simulink model "env_extQ16"  (R2022b)
settings: Solver=VariableStepAuto  StartTime=0.0  StopTime=30  RelTol=1e-3
values from neighbouring files (symbols this model uses):
  B = 8    [variables.m]    (also in variables16.m)
  cordic_delay = 20    [variables.m]    (also in variables16.m)
  e_val = 1/l2    [variables.m]    (also in variables16.m)
  exp_fract_len_homo = 26    [variables.m]    (also in variables16.m = 10)
  exp_word_len_homo = 32    [variables.m]    (also in variables16.m = 16)
  explarge_delay = 3    [variables.m]    (also in variables16.m)
  fft_len_hilb = 2048    [variables.m]    (also in variables16.m)
  fft_length = 4096    [variables.m]    (also in variables16.m)
  frac_bit_l2 = 30    [variables.m]    (also in variables16.m = 14)
  frac_bit_l3 = 29    [variables.m]    (also in variables16.m = 13)
  frac_bit_l4 = 28    [variables.m]    (also in variables16.m = 12)
  grp_delay_hilb = 11    [variables.m]    (also in variables16.m)
  grp_delay_homo = 13    [variables.m]    (also in variables16.m)
  grp_delay_psd = 19    [variables.m]    (also in variables16.m)
  grp_delay_swt = 12    [variables.m]    (also in variables16.m)
  l2 = log(2)    [variables.m]    (also in variables16.m)
  l2e = 1/log2(exp(1))    [variables.m]    (also in variables16.m)
  log2_table = log2((2^(B-1) : 2^(B)) / 2^(B - 1))    [variables.m]    (also in variables16.m)
  log_fract_len_homo = 31    [variables.m]    (also in variables16.m = 15)
  log_latency = 21    [variables.m]    (also in variables16.m)
  log_word_len = 48    [variables.m]    (also in variables16.m = 24)
  log_word_len_homo = 32    [variables.m]    (also in variables16.m = 16)
  NLZLUT = B-ceil(log2((1:2^B)))    [variables.m]    (also in variables16.m)
  scale = 1.0 / (fs * sum(window_val.*window_val))    [variables.m]    (also in variables16.m)
  win_dim = 64    [variables.m]    (also in variables16.m)
  window_dim = 100    [variables.m]    (also in variables16.m)
undefined symbols (not defined in the file or in its folder): C, c, fl_high_index, fl_low_index, HiD, hilbert_fifo_full, LoD, psd_fifo_full, SFVC784, swt_fifo_full, XCK26, xlfda_numerator
libraries: hdlBasic x626, hdlDSPIP x12, hdlUtilities x2, dspsnks4 x1, dspvision x1, vmcUtilities x1
(part 3 of 7)

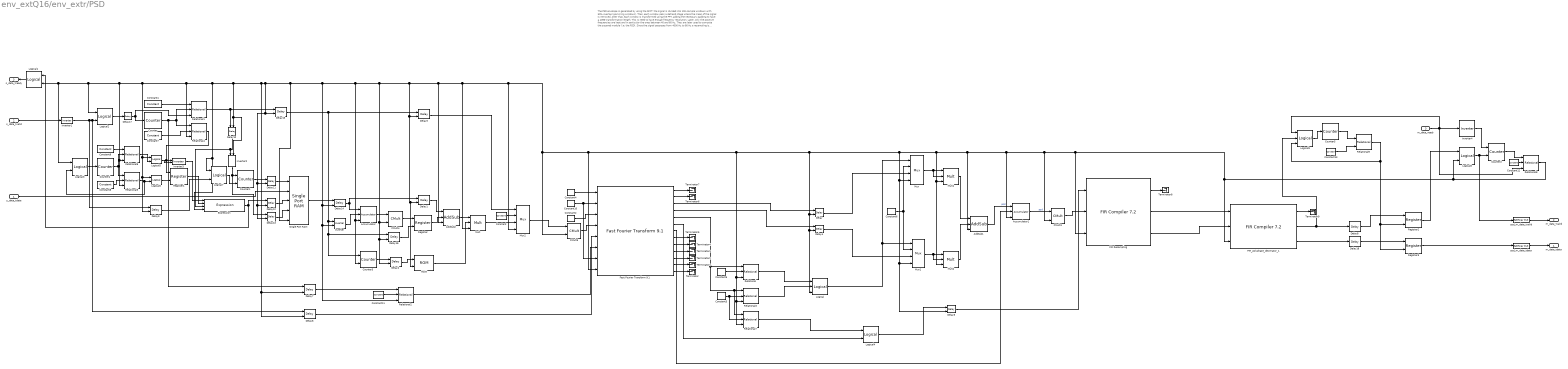
== system env_extQ16/env_extr/PSD ==
  note: The PSD envelope is generated by using the SFFT: the signal is divided into 100-sample windows with 50% overlap (Hamming windows). Then, each window pass a detrend stage where the mean of the signal is removed. After that, each window is transformed using the FFT, adding the necessary padding to have a 4096 transformation length. This is need to have enough frequency resolution.
      | Later, only the positive frequencies are kept and in particular the ones between 40 and 60 Hz. They are later used to compute the squared module (i.e. the PSD).
      | Since the signal passeses from 4000 Hz to 80 Hz a resampling is needed and instead of using a resample method based on FFT, a polyphase interpolator is employed.
      |
      | More at: https://docs.scipy.org/doc/scipy/reference/generated/scipy.signal.spectrogram.html and
      | https://ieeexplore.ieee.org/document/7234876
  s_data_tdata : Inport
  s_data_tvalid : Inport  Port=2
  m_data_ready : Inport  Port=3
  Accumulator : hdlBasic/Accumulator  operation=Add  n_bits=32  overflow=Wrap  scale=1  rst=on  hasbypass=off  en=on  latency=1  msb_inp=100  msb=100  lsb=-100  use_behavioral_HDL=on  implementation=Fabric  XmcBlockStatus=1  maskContainerNames=group3  block_type=accum  block_config=sysgen:Accum_config  block_width=566  block_height=845
  Accumulator1 : hdlBasic/Accumulator  operation=Add  n_bits=64  overflow=Wrap  scale=1  rst=on  hasbypass=off  en=on  latency=1  msb_inp=203  msb=203  lsb=-100  use_behavioral_HDL=on  implementation=Fabric  XmcBlockStatus=1  maskContainerNames=group3  block_type=accum  block_config=sysgen:Accum_config  block_width=566  block_height=845
  AddSub1 : hdlBasic/AddSub  mode=Addition  use_carryin=off  use_carryout=off  en=on  latency=1  precision=User Defined  arith_type="Signed  (2's comp)"  n_bits=32  bin_pt=30  quantization="Round  (unbiased: +/- Inf)"  overflow=Wrap  use_behavioral_HDL=off  hw_selection=Fabric  pipelined=off  XmcBlockStatus=1  maskContainerNames=tabcontainer1  block_type=addsub  block_config=sysgen:Addsub_config
  AddSub2 : hdlBasic/AddSub  mode=Subtraction  use_carryin=off  use_carryout=off  en=on  latency=1  precision=User Defined  arith_type="Signed  (2's comp)"  n_bits=32  bin_pt=31  quantization="Round  (unbiased: +/- Inf)"  overflow=Wrap  use_behavioral_HDL=off  hw_selection=Fabric  pipelined=off  XmcBlockStatus=1  maskContainerNames=tabcontainer1  block_type=addsub  block_config=sysgen:Addsub_config
  CMult3 : hdlBasic/CMult  const=(scale*128*128*2*2)/(fl_high_index-fl_low_index)  gui_display_data_type=Fixed-point  const_n_bits=32  const_bin_pt=31  float_type=Single  exp_bits=8  fraction_bits=24  en=on  latency=1  precision=User Defined  arith_type="Signed  (2's comp)"  n_bits=32  bin_pt=30  quantization="Round  (unbiased: +/- Inf)"  overflow=Wrap  use_behavioral_HDL=off  mem_type=Distributed RAM  pipeline=off  XmcBlockStatus=1  maskContainerNames=tabcontainer1  block_type=cmult  block_config=sysgen:CMult_config
      settings: infoedit=[]
  CMult4 : hdlBasic/CMult  const=1/window_dim  gui_display_data_type=Fixed-point  const_n_bits=32  const_bin_pt=31  float_type=Single  exp_bits=8  fraction_bits=24  en=on  latency=1  precision=User Defined  arith_type="Signed  (2's comp)"  n_bits=32  bin_pt=30  quantization="Round  (unbiased: +/- Inf)"  overflow=Wrap  use_behavioral_HDL=off  mem_type=Distributed RAM  pipeline=off  XmcBlockStatus=1  maskContainerNames=tabcontainer1  block_type=cmult  block_config=sysgen:CMult_config
      settings: infoedit=[]
  CMult5 : hdlBasic/CMult  const=1/128  gui_display_data_type=Fixed-point  const_n_bits=32  const_bin_pt=31  float_type=Single  exp_bits=8  fraction_bits=24  en=on  latency=1  precision=User Defined  arith_type="Signed  (2's comp)"  n_bits=32  bin_pt=31  quantization="Round  (unbiased: +/- Inf)"  overflow=Wrap  use_behavioral_HDL=off  mem_type=Distributed RAM  pipeline=off  XmcBlockStatus=1  maskContainerNames=tabcontainer1  block_type=cmult  block_config=sysgen:CMult_config
      settings: infoedit=[]
  Constant : hdlBasic/Constant  const=0  gui_display_data_type=Fixed-point  arith_type=Signed (2's comp)  n_bits=32  bin_pt=31  preci_type=Single  exp_width=8  frac_width=24  explicit_period=off  period=1  XmcBlockStatus=1  maskContainerNames=tabcontainer1  block_type=constant  block_config=sysgen:Constant_config
  Constant1 : hdlBasic/Constant  const=window_dim  gui_display_data_type=Fixed-point  arith_type=Unsigned  n_bits=ceil(log2(window_dim))  bin_pt=0  preci_type=Single  exp_width=8  frac_width=24  explicit_period=off  period=1  XmcBlockStatus=1  maskContainerNames=tabcontainer1  block_type=constant  block_config=sysgen:Constant_config
  Constant10 : hdlBasic/Constant  const=1.0  gui_display_data_type=Boolean  arith_type=Boolean  n_bits=16  bin_pt=14  preci_type=Single  exp_width=8  frac_width=24  explicit_period=off  period=1  XmcBlockStatus=1  maskContainerNames=tabcontainer1  block_type=constant  block_config=sysgen:Constant_config
  Constant11 : hdlBasic/Constant  const=4094  gui_display_data_type=Fixed-point  arith_type=Unsigned  n_bits=ceil(log2(fft_length))  bin_pt=0  preci_type=Single  exp_width=8  frac_width=24  explicit_period=off  period=1  XmcBlockStatus=1  maskContainerNames=tabcontainer1  block_type=constant  block_config=sysgen:Constant_config
  Constant12 : hdlBasic/Constant  const=win_dim  gui_display_data_type=Fixed-point  arith_type=Unsigned  n_bits=win_bit  bin_pt=0  preci_type=Single  exp_width=8  frac_width=24  explicit_period=off  period=1  XmcBlockStatus=1  maskContainerNames=tabcontainer1  block_type=constant  block_config=sysgen:Constant_config
  Constant13 : hdlBasic/Constant  const=grp_delay_psd  gui_display_data_type=Fixed-point  arith_type=Unsigned  n_bits=ceil(log2(grp_delay_psd))  bin_pt=0  preci_type=Single  exp_width=8  frac_width=24  explicit_period=off  period=1  XmcBlockStatus=1  maskContainerNames=tabcontainer1  block_type=constant  block_config=sysgen:Constant_config
  Constant2 : hdlBasic/Constant  const=0  gui_display_data_type=Fixed-point  arith_type=Signed (2's comp)  n_bits=32  bin_pt=31  preci_type=Single  exp_width=8  frac_width=24  explicit_period=on  period=sample_period_psd  XmcBlockStatus=1  maskContainerNames=tabcontainer1  block_type=constant  block_config=sysgen:Constant_config
  Constant3 : hdlBasic/Constant  const=fl_high_index-1  gui_display_data_type=Fixed-point  arith_type=Unsigned  n_bits=ceil(log2(fl_high_index-1))  bin_pt=0  preci_type=Single  exp_width=8  frac_width=24  explicit_period=off  period=1  XmcBlockStatus=1  maskContainerNames=tabcontainer1  block_type=constant  block_config=sysgen:Constant_config
  Constant4 : hdlBasic/Constant  const=1.0  gui_display_data_type=Fixed-point  arith_type=Unsigned  n_bits=1  bin_pt=0  preci_type=Single  exp_width=8  frac_width=24  explicit_period=off  period=1  XmcBlockStatus=1  maskContainerNames=tabcontainer1  block_type=constant  block_config=sysgen:Constant_config
  Constant5 : hdlBasic/Constant  const=fl_low_index-1  gui_display_data_type=Fixed-point  arith_type=Unsigned  n_bits=ceil(log2(fl_low_index-1))  bin_pt=0  preci_type=Single  exp_width=8  frac_width=24  explicit_period=off  period=1  XmcBlockStatus=1  maskContainerNames=tabcontainer1  block_type=constant  block_config=sysgen:Constant_config
  Constant6 : hdlBasic/Constant  const=0  gui_display_data_type=Fixed-point  arith_type=Signed (2's comp)  n_bits=32  bin_pt=30  preci_type=Single  exp_width=8  frac_width=24  explicit_period=off  period=1  XmcBlockStatus=1  maskContainerNames=tabcontainer1  block_type=constant  block_config=sysgen:Constant_config
  Constant7 : hdlBasic/Constant  const=(window_dim/2)-1  gui_display_data_type=Fixed-point  arith_type=Unsigned  n_bits=ceil(log2((window_dim/2)-1))  bin_pt=0  preci_type=Single  exp_width=8  frac_width=24  explicit_period=off  period=1  XmcBlockStatus=1  maskContainerNames=tabcontainer1  block_type=constant  block_config=sysgen:Constant_config
  Constant8 : hdlBasic/Constant  const=(window_dim/2)  gui_display_data_type=Fixed-point  arith_type=Unsigned  n_bits=ceil(log2((window_dim/2)+2))  bin_pt=0  preci_type=Single  exp_width=8  frac_width=24  explicit_period=off  period=1  XmcBlockStatus=1  maskContainerNames=tabcontainer1  block_type=constant  block_config=sysgen:Constant_config
  Constant9 : hdlBasic/Constant  const=(window_dim/2)-1  gui_display_data_type=Fixed-point  arith_type=Unsigned  n_bits=ceil(log2((window_dim/2)+1))  bin_pt=0  preci_type=Single  exp_width=8  frac_width=24  explicit_period=off  period=1  XmcBlockStatus=1  maskContainerNames=tabcontainer1  block_type=constant  block_config=sysgen:Constant_config
  Counter : hdlBasic/Counter  cnt_type=Free running  cnt_to=4094  operation=Up  start_count=0  cnt_by_val=1  arith_type=Unsigned  n_bits=ceil(log2(fft_length))  bin_pt=0  load_pin=off  rst=off  en=on  explicit_period=Explicit  period=sample_period_psd  use_behavioral_HDL=off  implementation=Fabric  XmcBlockStatus=1  maskContainerNames=group1  block_type=counter  block_config=sysgen:Counter_config  block_width=531  block_height=1023
  Counter1 : hdlBasic/Counter  cnt_type=Count limited  cnt_to=(window_dim/2)-1  operation=Up  start_count=0  cnt_by_val=1  arith_type=Unsigned  n_bits=ceil(log2((window_dim/2)-1))  bin_pt=0  load_pin=off  rst=on  en=on  explicit_period=Explicit  period=sample_period_psd  use_behavioral_HDL=off  implementation=Fabric  XmcBlockStatus=1  maskContainerNames=group1  block_type=counter  block_config=sysgen:Counter_config  block_width=531  block_height=1023
  Counter2 : hdlBasic/Counter  cnt_type=Free running  cnt_to=Inf  operation=Up  start_count=0  cnt_by_val=1  arith_type=Unsigned  n_bits=win_bit  bin_pt=0  load_pin=off  rst=on  en=on  explicit_period=Explicit  period=sample_period_psd  use_behavioral_HDL=off  implementation=Fabric  XmcBlockStatus=1  maskContainerNames=group1  block_type=counter  block_config=sysgen:Counter_config  block_width=531  block_height=1023
  Counter3 : hdlBasic/Counter  cnt_type=Count limited  cnt_to=window_dim-1  operation=Up  start_count=0  cnt_by_val=1  arith_type=Unsigned  n_bits=ceil(log2(window_dim-1))  bin_pt=0  load_pin=off  rst=on  en=on  explicit_period=Explicit  period=sample_period_psd  use_behavioral_HDL=off  implementation=Fabric  XmcBlockStatus=1  maskContainerNames=group1  block_type=counter  block_config=sysgen:Counter_config  block_width=531  block_height=1023
  Counter4 : hdlBasic/Counter  cnt_type=Free running  cnt_to=100  operation=Up  start_count=0  cnt_by_val=1  arith_type=Unsigned  n_bits=7  bin_pt=0  load_pin=off  rst=off  en=on  explicit_period=Explicit  period=sample_period_psd  use_behavioral_HDL=off  implementation=Fabric  XmcBlockStatus=1  maskContainerNames=group1  block_type=counter  block_config=sysgen:Counter_config  block_width=531  block_height=1023
  Counter5 : hdlBasic/Counter  cnt_type=Free running  cnt_to=Inf  operation=Up  start_count=0  cnt_by_val=1  arith_type=Unsigned  n_bits=ceil(log2(grp_delay_psd))  bin_pt=0  load_pin=off  rst=off  en=on  explicit_period=Explicit  period=sample_period_psd  use_behavioral_HDL=off  implementation=Fabric  XmcBlockStatus=1  maskContainerNames=group1  block_type=counter  block_config=sysgen:Counter_config  block_width=531  block_height=1023
  Delay : hdlBasic/Delay  rst=off  en=on  latency=2  reg_retiming=off  XmcBlockStatus=1  maskContainerNames=group1  block_type=delay  block_config=sysgen:Delay_config
  Delay1 : hdlBasic/Delay  rst=off  en=on  latency=window_dim+2  reg_retiming=off  XmcBlockStatus=1  maskContainerNames=group1  block_type=delay  block_config=sysgen:Delay_config
  Delay{10..14} (5 alike) : hdlBasic/Delay  rst=off  en=on  latency=1  reg_retiming=off  XmcBlockStatus=1  maskContainerNames=group1  block_type=delay  block_config=sysgen:Delay_config
  Delay15 : hdlBasic/Delay  rst=off  en=on  latency=4  reg_retiming=off  XmcBlockStatus=1  maskContainerNames=group1  block_type=delay  block_config=sysgen:Delay_config
  Delay16 : hdlBasic/Delay  rst=off  en=on  latency=3  reg_retiming=off  XmcBlockStatus=1  maskContainerNames=group1  block_type=delay  block_config=sysgen:Delay_config
  Delay17 : hdlBasic/Delay  rst=off  en=off  latency=1  reg_retiming=off  XmcBlockStatus=1  maskContainerNames=group1  block_type=delay  block_config=sysgen:Delay_config
  Delay18 : hdlBasic/Delay  rst=off  en=off  latency=1  reg_retiming=off  XmcBlockStatus=1  maskContainerNames=group1  block_type=delay  block_config=sysgen:Delay_config
  Delay2 : hdlBasic/Delay  rst=off  en=on  latency=3  reg_retiming=off  XmcBlockStatus=1  maskContainerNames=group1  block_type=delay  block_config=sysgen:Delay_config
  Delay3 : hdlBasic/Delay  rst=off  en=on  latency=window_dim+7  reg_retiming=off  XmcBlockStatus=1  maskContainerNames=group1  block_type=delay  block_config=sysgen:Delay_config
  Delay4 : hdlBasic/Delay  rst=off  en=on  latency=2  reg_retiming=off  XmcBlockStatus=1  maskContainerNames=group1  block_type=delay  block_config=sysgen:Delay_config
  Delay5 : hdlBasic/Delay  rst=off  en=on  latency=8  reg_retiming=off  XmcBlockStatus=1  maskContainerNames=group1  block_type=delay  block_config=sysgen:Delay_config
  Delay6 : hdlBasic/Delay  rst=off  en=on  latency=114  reg_retiming=off  XmcBlockStatus=1  maskContainerNames=group1  block_type=delay  block_config=sysgen:Delay_config
  Delay7 : hdlBasic/Delay  rst=off  en=on  latency=113  reg_retiming=off  XmcBlockStatus=1  maskContainerNames=group1  block_type=delay  block_config=sysgen:Delay_config
  Delay8 : hdlBasic/Delay  rst=off  en=off  latency=1  reg_retiming=off  XmcBlockStatus=1  maskContainerNames=group1  block_type=delay  block_config=sysgen:Delay_config
  Delay9 : hdlBasic/Delay  rst=off  en=on  latency=3  reg_retiming=off  XmcBlockStatus=1  maskContainerNames=group1  block_type=delay  block_config=sysgen:Delay_config
  Expression : hdlBasic/Expression  expression=~(a ^ b) & c  align_bp=on  en=on  latency=1  precision=Full  arith_type=Unsigned  n_bits=16  bin_pt=0  XmcBlockStatus=1  maskContainerNames=tabcontainer1  block_type=expr  block_config=sysgen:Expr_config
  FIR Resampling : hdlDSPIP/FIR Compiler 7.2   coefficientvector=fir_interpolator.Numerator  coefficient_sets=1  coefficient_reload=off  filter_type=Interpolation  rate_change_type=Integer  interpolation_rate=50  decimation_rate=1  zero_pack_factor=1  channel_sequence=Basic  number_channels=1  pattern_list='P4-0,P4-1,P4-2,P4-3,P4-4'  number_paths=1  ratespecification=Input_Sample_Period  sampleperiod=fft_length  hardwareoversamplingrate=1  coefficient_sign=Signed  quantization=Quantize_Only  coefficient_width=coeff_width  bestprecision=on  coefficient_fractional_bits=30  coefficient_structure=Non_Symmetric  output_rounding_mode=Convergent_Rounding_to_Even  output_width=output_width  filter_architecture=Systolic_Multiply_Accumulate  optimization_goal=Area  optimization_list='None'  data_buffer_type=Automatic  coefficient_buffer_type=Automatic  input_buffer_type=Automatic  output_buffer_type=Automatic  preference_for_other_storage=Automatic  multi_column_support=Automatic  columnconfig='1'  inter_column_pipe_length=4  data_has_tlast=Not_Required  m_data_has_tready=off  s_data_has_fifo=off  s_data_has_tuser=Not_Required  m_data_has_tuser=Not_Required  s_config_sync_mode=On_Vector  s_config_method=Single  num_reload_slots=1  has_aclken=on  has_aresetn=off  reset_data_vector=on  trim_axipin_name=off  simulation_type=hybrid_sim  simulation_model=sysgen:xfirv7_2_cmodel  data_path_portlist={ 's_axis_data_tdata', 'm_axis_data_tdata' }  passband_min=0.0  passband_max=0.5  stopband_min=0.5  stopband_max=1.0  filter_selection=1  gui_behaviour='Sysgen_GUI'  data_sign=Signed  data_width=16  data_fractional_bits=0  data_tuser_width=1  wrapper_available=true  ip_wrap_arbitrary_binary_point=true  ip_name=FIR Compiler  ip_version=7.2  dsptool_ready=true  ipcore_usecache=true  ipcore_useipmodelcache=true  port_translation_map={ 'aclken' => 'en', 'aresetn' => 'rst' }  run_core_at_system_period=true  ipcore_xco_need_fpga_part=true  ipcore_fpga_part=[]  XmcBlockStatus=1  maskContainerNames=tabcontainer1  block_type=fir_compiler_v7_2  block_config=sysgen:rodinimport_config  block_width=820  block_height=600
  FIR_polyphase_decimator_1 : hdlDSPIP/FIR Compiler 7.2   coefficientvector=firdecim.Numerator  coefficient_sets=1  coefficient_reload=off  filter_type=Decimation  rate_change_type=Integer  interpolation_rate=1  decimation_rate=80  zero_pack_factor=1  channel_sequence=Basic  number_channels=1  pattern_list='P4-0,P4-1,P4-2,P4-3,P4-4'  number_paths=1  ratespecification=Input_Sample_Period  sampleperiod=1  hardwareoversamplingrate=1  coefficient_sign=Signed  quantization=Quantize_Only  coefficient_width=coeff_width  bestprecision=on  coefficient_fractional_bits=37  coefficient_structure=Non_Symmetric  output_rounding_mode=Convergent_Rounding_to_Even  output_width=output_width  filter_architecture=Systolic_Multiply_Accumulate  optimization_goal=Area  optimization_list='None'  data_buffer_type=Automatic  coefficient_buffer_type=Automatic  input_buffer_type=Automatic  output_buffer_type=Automatic  preference_for_other_storage=Automatic  multi_column_support=Automatic  columnconfig='24'  inter_column_pipe_length=4  data_has_tlast=Not_Required  m_data_has_tready=off  s_data_has_fifo=off  s_data_has_tuser=Not_Required  m_data_has_tuser=Not_Required  s_config_sync_mode=On_Vector  s_config_method=Single  num_reload_slots=1  has_aclken=on  has_aresetn=off  reset_data_vector=on  trim_axipin_name=off  simulation_type=hybrid_sim  simulation_model=sysgen:xfirv7_2_cmodel  data_path_portlist={ 's_axis_data_tdata', 'm_axis_data_tdata' }  passband_min=0.0  passband_max=0.5  stopband_min=0.5  stopband_max=1.0  filter_selection=1  gui_behaviour='Sysgen_GUI'  data_sign=Signed  data_width=16  data_fractional_bits=0  data_tuser_width=1  wrapper_available=true  ip_wrap_arbitrary_binary_point=true  ip_name=FIR Compiler  ip_version=7.2  dsptool_ready=true  ipcore_usecache=true  ipcore_useipmodelcache=true  port_translation_map={ 'aclken' => 'en', 'aresetn' => 'rst' }  run_core_at_system_period=true  ipcore_xco_need_fpga_part=true  ipcore_fpga_part=[]  XmcBlockStatus=1  maskContainerNames=tabcontainer1  block_type=fir_compiler_v7_2  block_config=sysgen:rodinimport_config  block_width=820  block_height=600
  Fast Fourier Transform 9.1 : hdlDSPIP/Fast Fourier Transform 9.1   transform_length=4096  target_clock_frequency=fft_freq_psd  target_data_throughput=50  implementation_options=pipelined_streaming_io  run_time_configurable_transform_length=off  phase_factor_width=32  scaling_options=unscaled  rounding_modes=convergent_rounding  aclken=on  aresetn=off  output_ordering=natural_order  cyclic_prefix_insertion=off  throttle_scheme=nonrealtime  xk_index=on  ovflo=off  trim_axipin_name=off  memory_options_data=block_ram  memory_options_phase_factors=block_ram  number_of_stages_using_block_ram_for_data_and_phase_factors=6  memory_options_reorder=block_ram  memory_options_hybrid=off  complex_mult_type=use_mults_resources  butterfly_type=use_luts  simulation_type=hybrid_sim  simulation_model=sysgen:xfftv9_cmodel  data_path_portlist={ 's_axis_data_tdata', 'm_axis_data_tdata', 'm_axis_status_tdata', 'event_fft_overflow' }  channels=1  input_ordering=natural_order  input_width=16  ip_name=Fast Fourier Transform  ip_version=9.1  dsptool_ready=true  ipcore_usecache=true  ipcore_useipmodelcache=true  wrapper_available=true  port_translation_map={ 'aclken' => 'en', 'aresetn' => 'rst'}  data_format=fixed_point  XmcBlockStatus=1  maskContainerNames=tabcontainer1  block_type=xfft_v9_1  block_config=sysgen:rodinimport_config
  Inverter : hdlBasic/Inverter  en=on  latency=1  XmcBlockStatus=1  maskContainerNames=group2  block_type=inv  block_config=sysgen:Inverter_config
  Inverter1 : hdlBasic/Inverter  en=off  latency=0  XmcBlockStatus=1  maskContainerNames=group2  block_type=inv  block_config=sysgen:Inverter_config
  Inverter2 : hdlBasic/Inverter  en=on  latency=1  XmcBlockStatus=1  maskContainerNames=group2  block_type=inv  block_config=sysgen:Inverter_config
  Inverter3 : hdlBasic/Inverter  en=on  latency=1  XmcBlockStatus=1  maskContainerNames=group2  block_type=inv  block_config=sysgen:Inverter_config
  Inverter4 : hdlBasic/Inverter  en=off  latency=0  XmcBlockStatus=1  maskContainerNames=group2  block_type=inv  block_config=sysgen:Inverter_config
  Logical : hdlBasic/Logical  logical_function=AND  inputs=2  en=on  latency=1  precision=Full  arith_type=Unsigned  n_bits=16  bin_pt=0  align_bp=on  overflow=[]  quantization=[]  XmcBlockStatus=1  maskContainerNames=tabcontainer1  block_type=logical  block_config=sysgen:Logical_config
  Logical{1..8} (8 alike) : hdlBasic/Logical  logical_function=AND  inputs=2  en=off  latency=0  precision=Full  arith_type=Unsigned  n_bits=16  bin_pt=0  align_bp=on  overflow=[]  quantization=[]  XmcBlockStatus=1  maskContainerNames=tabcontainer1  block_type=logical  block_config=sysgen:Logical_config
  Logical9 : hdlBasic/Logical  logical_function=AND  inputs=3  en=off  latency=0  precision=Full  arith_type=Unsigned  n_bits=16  bin_pt=0  align_bp=on  overflow=[]  quantization=[]  XmcBlockStatus=1  maskContainerNames=tabcontainer1  block_type=logical  block_config=sysgen:Logical_config
  Mult : hdlBasic/Mult  precision=User Defined  arith_type="Signed  (2's comp)"  n_bits=32  bin_pt=31  quantization="Round  (unbiased: +/- Inf)"  overflow=Wrap  en=on  latency=3  use_behavioral_HDL=off  opt=Speed  use_embedded=on  optimum_pipeline=off  pipeline=on  use_rpm=on  placement_style=Triangular  XmcBlockStatus=1  maskContainerNames=group1  block_type=mult  block_config=sysgen:Mult_config  block_width=598  block_height=876
  Mult1 : hdlBasic/Mult  precision=User Defined  arith_type="Signed  (2's comp)"  n_bits=32  bin_pt=30  quantization="Round  (unbiased: +/- Inf)"  overflow=Wrap  en=on  latency=3  use_behavioral_HDL=off  opt=Speed  use_embedded=on  optimum_pipeline=off  pipeline=on  use_rpm=on  placement_style=Triangular  XmcBlockStatus=1  maskContainerNames=group1  block_type=mult  block_config=sysgen:Mult_config  block_width=598  block_height=876
  Mult2 : hdlBasic/Mult  precision=User Defined  arith_type="Signed  (2's comp)"  n_bits=32  bin_pt=30  quantization="Round  (unbiased: +/- Inf)"  overflow=Wrap  en=on  latency=3  use_behavioral_HDL=off  opt=Speed  use_embedded=on  optimum_pipeline=off  pipeline=on  use_rpm=on  placement_style=Triangular  XmcBlockStatus=1  maskContainerNames=group1  block_type=mult  block_config=sysgen:Mult_config  block_width=598  block_height=876
  Mux : hdlBasic/Mux  inputs=2  en=on  latency=1  precision=Full  arith_type=Unsigned  n_bits=16  bin_pt=14  quantization=Truncate  overflow=Wrap  XmcBlockStatus=1  maskContainerNames=tabcontainer1  block_type=mux  block_config=sysgen:Mux_config
  Mux1 : hdlBasic/Mux  inputs=2  en=on  latency=1  precision=Full  arith_type=Unsigned  n_bits=16  bin_pt=14  quantization=Truncate  overflow=Wrap  XmcBlockStatus=1  maskContainerNames=tabcontainer1  block_type=mux  block_config=sysgen:Mux_config
  Mux2 : hdlBasic/Mux  inputs=2  en=on  latency=1  precision=Full  arith_type="Signed  (2's comp)"  n_bits=32  bin_pt=28  quantization="Round  (unbiased: +/- Inf)"  overflow=Wrap  XmcBlockStatus=1  maskContainerNames=tabcontainer1  block_type=mux  block_config=sysgen:Mux_config
  ROM : hdlBasic/ROM  depth=window_dim  initVector=window_val  distributed_mem=Block RAM  rst=off  init_reg=0  en=on  latency=1  gui_display_data_type=Fixed-point  arith_type="Signed  (2's comp)"  n_bits=32  bin_pt=31  preci_type=Single  exp_width=8  frac_width=24  optimize=Area  use_rpm=on  simulation_type=fast_sim  XmcBlockStatus=1  maskContainerNames=tabcontainer1  block_type=sprom  block_config=sysgen:SPROM_config
  Register : hdlBasic/Register  init=0  rst=off  en=on  XmcBlockStatus=1  maskContainerNames=tabcontainer1  block_type=register  block_config=sysgen:Register_config
  Register1 : hdlBasic/Register  init=0  rst=off  en=on  XmcBlockStatus=1  maskContainerNames=tabcontainer1  block_type=register  block_config=sysgen:Register_config
  Register2 : hdlBasic/Register  init=0  rst=on  en=off  XmcBlockStatus=1  maskContainerNames=tabcontainer1  block_type=register  block_config=sysgen:Register_config
  Register3 : hdlBasic/Register  init=0  rst=on  en=off  XmcBlockStatus=1  maskContainerNames=tabcontainer1  block_type=register  block_config=sysgen:Register_config
  Relational : hdlBasic/Relational  mode=a>=b  op_type=Bool  en=on  latency=1  XmcBlockStatus=1  maskContainerNames=tabcontainer1  block_type=relational  block_config=sysgen:Relational_config
  Relational1 : hdlBasic/Relational  mode=a>b  op_type=Bool  en=on  latency=1  XmcBlockStatus=1  maskContainerNames=tabcontainer1  block_type=relational  block_config=sysgen:Relational_config
  Relational2 : hdlBasic/Relational  mode=a=b  op_type=Bool  en=on  latency=1  XmcBlockStatus=1  maskContainerNames=tabcontainer1  block_type=relational  block_config=sysgen:Relational_config
  Relational3 : hdlBasic/Relational  mode=a<=b  op_type=Bool  en=on  latency=1  XmcBlockStatus=1  maskContainerNames=tabcontainer1  block_type=relational  block_config=sysgen:Relational_config
  Relational4 : hdlBasic/Relational  mode=a>b  op_type=Bool  en=on  latency=1  XmcBlockStatus=1  maskContainerNames=tabcontainer1  block_type=relational  block_config=sysgen:Relational_config
  Relational5 : hdlBasic/Relational  mode=a<b  op_type=Bool  en=on  latency=1  XmcBlockStatus=1  maskContainerNames=tabcontainer1  block_type=relational  block_config=sysgen:Relational_config
  Relational6 : hdlBasic/Relational  mode=a<b  op_type=Bool  en=on  latency=1  XmcBlockStatus=1  maskContainerNames=tabcontainer1  block_type=relational  block_config=sysgen:Relational_config
  Relational7 : hdlBasic/Relational  mode=a=b  op_type=Bool  en=on  latency=1  XmcBlockStatus=1  maskContainerNames=tabcontainer1  block_type=relational  block_config=sysgen:Relational_config
  Relational8 : hdlBasic/Relational  mode=a<b  op_type=Bool  en=on  latency=1  XmcBlockStatus=1  maskContainerNames=tabcontainer1  block_type=relational  block_config=sysgen:Relational_config
  Relational9 : hdlBasic/Relational  mode=a<b  op_type=Bool  en=off  latency=0  XmcBlockStatus=1  maskContainerNames=tabcontainer1  block_type=relational  block_config=sysgen:Relational_config
  Single Port RAM : hdlBasic/Single Port RAM  depth=window_dim/2  initVector=zeros(1,window_dim/2)  distributed_mem=Block RAM  write_mode=Read After Write  rst=on  init_reg=0  en=on  optimize_latency=off  latency=1  optimize=Area  dbl_ovrd=off  simulation_type=fast_sim  XmcBlockStatus=1  maskContainerNames=tabcontainer1  block_type=spram  block_config=sysgen:SPRAM_config
  Terminator{,1..9} (10 alike) : Terminator
  psd_m_data_tdata : hdlBasic/Gateway Out  inherit_from_input=off  hdl_port=on  rows=1  columns=1  UseAsDAC=off  DACChannel='1'  interface=None  automatic_assignment=on  address_offset=hex2dec('00')  intf_name=''  intf_description=''  timing_constraint=None  locs_specified=off  LOCs={}  io_standard={}  XmcBlockStatus=1  maskContainerNames=group4  block_type=gatewayout  block_config=sysgen:gateway_out_config  block_width_w=590  block_height_w=620  block_width=620  block_height=750
  psd_m_data_tvalid : hdlBasic/Gateway Out  inherit_from_input=off  hdl_port=on  rows=1  columns=1  UseAsDAC=off  DACChannel='1'  interface=None  automatic_assignment=on  address_offset=hex2dec('00')  intf_name=''  intf_description=''  timing_constraint=None  locs_specified=off  LOCs={}  io_standard={}  XmcBlockStatus=1  maskContainerNames=group4  block_type=gatewayout  block_config=sysgen:gateway_out_config  block_width_w=590  block_height_w=620  block_width=620  block_height=750
  m_data_tdata : Outport
  m_data_tvalid : Outport  Port=2
  s_data_tready : Outport  Port=3
  wires:
  Constant1/1 -> Relational1/1
  Mult/1 -> Mux2/3
  Constant8/1 -> Relational5/2
  Counter4/1 -> Relational6/2, Relational5/1
  Counter1/1 -> Delay11/1
  Accumulator1/1 -> CMult3/1  "psd"
  Delay2/1 -> ROM/1
  Relational/1 -> Logical/1
  Delay13/1 -> Single Port RAM/4
  Accumulator/1 -> CMult4/1
  Delay16/1 -> Register/2
  Delay10/1 -> Expression/3, Inverter2/1
  Counter3/1 -> Delay2/1
  Delay14/1 -> Delay1/1, Accumulator/1
  Single Port RAM/1 -> Delay14/1
  Relational1/1 -> Delay15/1, Delay10/1
  Inverter3/1 -> Expression/1
  Constant/1 -> Mux2/2
  Delay3/1 -> Mux2/1
  Delay15/1 -> Delay3/1, Counter3/1, Delay16/1, Inverter/1
  Constant6/1 -> Mux1/2, Mux/2
  CMult4/1 -> Register/1
  Mux2/1 -> CMult5/1
  Inverter/1 -> Accumulator/2
  Constant9/1 -> Relational6/1
  Delay11/1 -> Single Port RAM/1
  Register1/1 -> Expression/2
  Constant7/1 -> Relational4/2
  Inverter2/1 -> Delay13/1, Counter1/1
  Relational4/1 -> Register1/1, Inverter3/1
  Expression/1 -> Delay12/1, Logical1/1
  AddSub2/1 -> Mult/1
  s_data_tdata/1 -> Single Port RAM/2
  Constant3/1 -> Relational7/2, Relational3/2
  s_data_tvalid/1 -> Inverter1/1
  Constant5/1 -> Relational/2
  Delay/1 -> Mux/3
  Mult1/1 -> AddSub1/1
  ROM/1 -> Mult/2
  Inverter1/1 -> Delay9/1, Delay6/1, Logical2/2
  Relational5/1 -> Logical6/2, Logical3/2
  Logical/1 -> Mux/1, Mux1/1
  Mult2/1 -> AddSub1/2
  Delay5/1 -> FIR Resampling/1
  Fast Fourier Transform 9.1/5 -> Relational/1, Relational7/1, Relational3/1
  Mux/1 -> Mult1/2, Mult1/1
  Delay4/1 -> Mux1/3
  Counter/1 -> Delay7/1, Relational4/1, Relational1/2
  Register/1 -> AddSub2/2
  AddSub1/1 -> Accumulator1/1  "psd"
  Delay1/1 -> AddSub2/1
  Mux1/1 -> Mult2/2, Mult2/1
  Relational3/1 -> Logical/2
  psd_m_data_tdata/1 -> m_data_tdata/1
  FIR Resampling/3 -> FIR_polyphase_decimator_1/2
  Fast Fourier Transform 9.1/13 -> Terminator/1
  Fast Fourier Transform 9.1/12 -> Terminator1/1
  Fast Fourier Transform 9.1/11 -> Terminator2/1
  Fast Fourier Transform 9.1/10 -> Terminator3/1
  Fast Fourier Transform 9.1/9 -> Terminator4/1
  Fast Fourier Transform 9.1/8 -> Terminator5/1
  Fast Fourier Transform 9.1/1 -> Terminator7/1
  Constant4/1 -> Fast Fourier Transform 9.1/1
  Constant10/1 -> Fast Fourier Transform 9.1/7, Fast Fourier Transform 9.1/2
  Constant2/1 -> Fast Fourier Transform 9.1/3
  Fast Fourier Transform 9.1/7 -> Accumulator1/2
  Fast Fourier Transform 9.1/3 -> Delay/1
  Fast Fourier Transform 9.1/4 -> Delay4/1
  CMult5/1 -> Fast Fourier Transform 9.1/4
  Logical1/1 -> s_data_tready/1
  Fast Fourier Transform 9.1/2 -> Terminator6/1
  Logical2/1 -> Delay17/1
  Logical3/1 -> Counter4/1
  Relational2/1 -> Fast Fourier Transform 9.1/6
  Constant11/1 -> Relational2/2
  Delay6/1 -> Fast Fourier Transform 9.1/5
  Delay7/1 -> Relational2/1
  Fast Fourier Transform 9.1/6 -> Logical4/2
  Logical4/1 -> Delay5/1
  Relational7/1 -> Logical4/1
  CMult3/1 -> FIR Resampling/2
  FIR Resampling/2 -> FIR_polyphase_decimator_1/1
  m_data_ready/1 -> Logical9/1, Relational8/3, Inverter4/1
  Delay9/1 -> Logical7/2
  Logical7/1 -> Counter1/2
  FIR Resampling/1 -> Terminator8/1
  FIR_polyphase_decimator_1/1 -> Terminator9/1
  Logical5/1 -> Inverter3/2
  Relational6/1 -> Logical5/2
  Logical6/1 -> Register1/2
  Delay17/1 -> Relational1/3, Counter/1
  Counter2/1 -> Relational8/1
  Constant12/1 -> Relational8/2
  Inverter4/1 -> Counter2/1
  Logical8/1 -> psd_m_data_tvalid/1, Counter2/2
  psd_m_data_tvalid/1 -> m_data_tvalid/1
  Relational8/1 -> FIR_polyphase_decimator_1/3, FIR Resampling/3, CMult3/2, Accumulator1/3, AddSub1/3, Mult2/3, Mult1/3, Delay5/2, Mux1/4, Mux/4, Logical/3, Delay4/2, Delay/2, Mux2/4, Mult/3, AddSub2/3, ROM/2, Delay1/2, Delay3/2, Delay2/2, Delay16/2, CMult4/2, Counter3/2, Accumulator/3, Relational2/3, Inverter/2, Delay14/2, Single Port RAM/5, Delay13/2, Delay12/2, Delay11/2, Delay15/2, Inverter2/2, Delay10/2, Logical7/1, Expression/4, Relational4/3, Logical5/1, Logical6/1, Delay9/2, Logical2/1, Logical3/1, Logical1/2, Relational5/3, Relational6/3, Delay6/2, Delay7/2, CMult5/2, Fast Fourier Transform 9.1/8, Relational3/3, Relational7/3, Relational/3, Logical8/2
  Delay12/1 -> Single Port RAM/3
  Counter5/1 -> Relational9/1
  Logical9/1 -> Counter5/1
  Relational9/1 -> Logical9/3, Register3/2, Register2/2
  Constant13/1 -> Relational9/2
  FIR_polyphase_decimator_1/3 -> Delay18/1
  FIR_polyphase_decimator_1/2 -> Logical9/2, Delay8/1
  Delay8/1 -> Register2/1
  Delay18/1 -> Register3/1
  Register2/1 -> Logical8/1
  Register3/1 -> psd_m_data_tdata/1

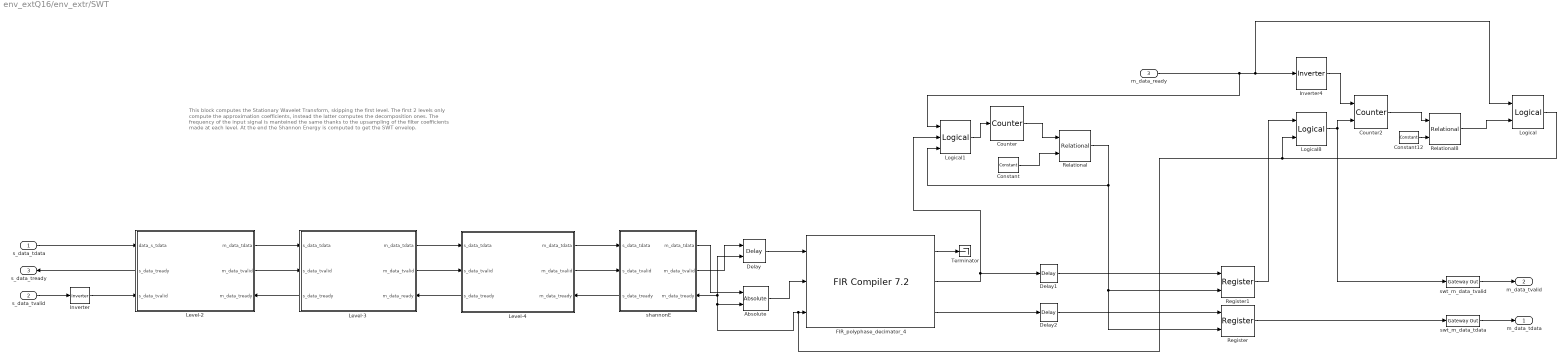
== system env_extQ16/env_extr/SWT ==
  note: This block computes the Stationary Wavelet Transform, skipping the first level. The first 2 levels only compute the approximation coefficients, instead the latter computes the decomposition ones.
      | The frequency of the input signal is manteined the same thanks to the upsampling of the filter coefficients made at each level. At the end the Shannon Energy is computed to get the SWT envelop.
  s_data_tdata : Inport
  s_data_tvalid : Inport  Port=2
  m_data_ready : Inport  Port=3
  Absolute : hdlBasic/Absolute  precision=User Defined  arith_type="Signed  (2's comp)"  n_bits=32  bin_pt=25  quantization="Round  (unbiased: +/- Inf)"  overflow=Saturate  en=on  latency=1  XmcBlockStatus=1  maskContainerNames=tabcontainer1  block_type=abs  block_config=sysgen:Abs_config
  Constant : hdlBasic/Constant  const=grp_delay_swt  gui_display_data_type=Fixed-point  arith_type=Unsigned  n_bits=ceil(log2(grp_delay_swt))  bin_pt=0  preci_type=Single  exp_width=8  frac_width=24  explicit_period=off  period=1  XmcBlockStatus=1  maskContainerNames=tabcontainer1  block_type=constant  block_config=sysgen:Constant_config
  Constant12 : hdlBasic/Constant  const=win_dim  gui_display_data_type=Fixed-point  arith_type=Unsigned  n_bits=win_bit  bin_pt=0  preci_type=Single  exp_width=8  frac_width=24  explicit_period=off  period=1  XmcBlockStatus=1  maskContainerNames=tabcontainer1  block_type=constant  block_config=sysgen:Constant_config
  Counter : hdlBasic/Counter  cnt_type=Free running  cnt_to=Inf  operation=Up  start_count=0  cnt_by_val=1  arith_type=Unsigned  n_bits=ceil(log2(grp_delay_swt))  bin_pt=0  load_pin=off  rst=off  en=on  explicit_period=Explicit  period=sample_period_swt  use_behavioral_HDL=off  implementation=Fabric  XmcBlockStatus=1  maskContainerNames=group1  block_type=counter  block_config=sysgen:Counter_config  block_width=531  block_height=1023
  Counter2 : hdlBasic/Counter  cnt_type=Free running  cnt_to=Inf  operation=Up  start_count=0  cnt_by_val=1  arith_type=Unsigned  n_bits=win_bit  bin_pt=0  load_pin=off  rst=on  en=on  explicit_period=Explicit  period=sample_period_swt  use_behavioral_HDL=off  implementation=Fabric  XmcBlockStatus=1  maskContainerNames=group1  block_type=counter  block_config=sysgen:Counter_config  block_width=531  block_height=1023
  Delay : hdlBasic/Delay  rst=off  en=on  latency=1  reg_retiming=off  XmcBlockStatus=1  maskContainerNames=group1  block_type=delay  block_config=sysgen:Delay_config
  Delay1 : hdlBasic/Delay  rst=off  en=off  latency=1  reg_retiming=off  XmcBlockStatus=1  maskContainerNames=group1  block_type=delay  block_config=sysgen:Delay_config
  Delay2 : hdlBasic/Delay  rst=off  en=off  latency=1  reg_retiming=off  XmcBlockStatus=1  maskContainerNames=group1  block_type=delay  block_config=sysgen:Delay_config
  FIR_polyphase_decimator_4 : hdlDSPIP/FIR Compiler 7.2   coefficientvector=firdecim.Numerator  coefficient_sets=1  coefficient_reload=off  filter_type=Decimation  rate_change_type=Integer  interpolation_rate=1  decimation_rate=80  zero_pack_factor=1  channel_sequence=Basic  number_channels=1  pattern_list='P4-0,P4-1,P4-2,P4-3,P4-4'  number_paths=1  ratespecification=Input_Sample_Period  sampleperiod=1  hardwareoversamplingrate=1  coefficient_sign=Signed  quantization=Quantize_Only  coefficient_width=coeff_width  bestprecision=on  coefficient_fractional_bits=21  coefficient_structure=Non_Symmetric  output_rounding_mode=Convergent_Rounding_to_Even  output_width=output_width  filter_architecture=Systolic_Multiply_Accumulate  optimization_goal=Area  optimization_list='None'  data_buffer_type=Automatic  coefficient_buffer_type=Automatic  input_buffer_type=Automatic  output_buffer_type=Automatic  preference_for_other_storage=Automatic  multi_column_support=Automatic  columnconfig='24'  inter_column_pipe_length=4  data_has_tlast=Not_Required  m_data_has_tready=off  s_data_has_fifo=off  s_data_has_tuser=Not_Required  m_data_has_tuser=Not_Required  s_config_sync_mode=On_Vector  s_config_method=Single  num_reload_slots=1  has_aclken=on  has_aresetn=off  reset_data_vector=on  trim_axipin_name=off  simulation_type=hybrid_sim  simulation_model=sysgen:xfirv7_2_cmodel  data_path_portlist={ 's_axis_data_tdata', 'm_axis_data_tdata' }  passband_min=0.0  passband_max=0.5  stopband_min=0.5  stopband_max=1.0  filter_selection=1  gui_behaviour='Sysgen_GUI'  data_sign=Signed  data_width=16  data_fractional_bits=0  data_tuser_width=1  wrapper_available=true  ip_wrap_arbitrary_binary_point=true  ip_name=FIR Compiler  ip_version=7.2  dsptool_ready=true  ipcore_usecache=true  ipcore_useipmodelcache=true  port_translation_map={ 'aclken' => 'en', 'aresetn' => 'rst' }  run_core_at_system_period=true  ipcore_xco_need_fpga_part=true  ipcore_fpga_part=[]  XmcBlockStatus=1  maskContainerNames=tabcontainer1  block_type=fir_compiler_v7_2  block_config=sysgen:rodinimport_config  block_width=820  block_height=600
  Inverter : hdlBasic/Inverter  en=off  latency=0  XmcBlockStatus=1  maskContainerNames=group2  block_type=inv  block_config=sysgen:Inverter_config
  Inverter4 : hdlBasic/Inverter  en=off  latency=0  XmcBlockStatus=1  maskContainerNames=group2  block_type=inv  block_config=sysgen:Inverter_config
  Level-2 : Subsystem
      settings: PortSchema="{\"entries\":[{\"content\":{\"sides\":[{\"content\":{\"connectorIds\":[\"In1\",\"Out3\",\"In2\"]},\"type\":\"ConnectorPlacement.EquallySpacedRectSide\",\"uuid\":\"9d039a16-3a48-49d5-80b7-ade04a8e7f96\"},{\"content\":{\"connectorIds\":[\"Out1\",\"Out2\",\"In3\"],\"side\":\"RIGHT\"},\"type\":\"ConnectorPlacement.EquallySpacedRectSide\",\"uuid\":\"bb4be220-296c-4d2d-b90e-a958a467eb47\"},{\"content\":{\"connectorIds\":[],\"side\":\"TOP\"},\"type\":\"ConnectorPlacement.EquallySpacedRectSide\",\"uuid\":\"bb4a24ca-25c4-4b34-8f6b-74df8c85655a\"}]},\"type\":\"ConnectorPlacement.EquallySpacedConnector\",\"uuid\":\"a2ca7259-7cd6-4f5b-b082-7ba40fce56a8\"}],\"packageUris\":[\"http://schema.mathworks.com/mf0/Connector/R2020b\"],\"version\":\"1.0\"}"
  Level-3 : Subsystem
      settings: PortSchema="{\"entries\":[{\"content\":{\"sides\":[{\"content\":{\"connectorIds\":[\"In1\",\"In2\",\"Out3\"]},\"type\":\"ConnectorPlacement.EquallySpacedRectSide\",\"uuid\":\"9d039a16-3a48-49d5-80b7-ade04a8e7f96\"},{\"content\":{\"connectorIds\":[\"Out1\",\"Out2\",\"In3\"],\"side\":\"RIGHT\"},\"type\":\"ConnectorPlacement.EquallySpacedRectSide\",\"uuid\":\"bb4be220-296c-4d2d-b90e-a958a467eb47\"},{\"content\":{\"connectorIds\":[],\"side\":\"TOP\"},\"type\":\"ConnectorPlacement.EquallySpacedRectSide\",\"uuid\":\"bb4a24ca-25c4-4b34-8f6b-74df8c85655a\"}]},\"type\":\"ConnectorPlacement.EquallySpacedConnector\",\"uuid\":\"a2ca7259-7cd6-4f5b-b082-7ba40fce56a8\"}],\"packageUris\":[\"http://schema.mathworks.com/mf0/Connector/R2020b\"],\"version\":\"1.0\"}"
  Level-4 : Subsystem
      settings: PortSchema="{\"entries\":[{\"content\":{\"sides\":[{\"content\":{\"connectorIds\":[\"In1\",\"In2\",\"Out3\"]},\"type\":\"ConnectorPlacement.EquallySpacedRectSide\",\"uuid\":\"9d039a16-3a48-49d5-80b7-ade04a8e7f96\"},{\"content\":{\"connectorIds\":[\"Out1\",\"Out2\",\"In3\"],\"side\":\"RIGHT\"},\"type\":\"ConnectorPlacement.EquallySpacedRectSide\",\"uuid\":\"bb4be220-296c-4d2d-b90e-a958a467eb47\"},{\"content\":{\"connectorIds\":[],\"side\":\"TOP\"},\"type\":\"ConnectorPlacement.EquallySpacedRectSide\",\"uuid\":\"bb4a24ca-25c4-4b34-8f6b-74df8c85655a\"}]},\"type\":\"ConnectorPlacement.EquallySpacedConnector\",\"uuid\":\"a2ca7259-7cd6-4f5b-b082-7ba40fce56a8\"}],\"packageUris\":[\"http://schema.mathworks.com/mf0/Connector/R2020b\"],\"version\":\"1.0\"}"
  Logical : hdlBasic/Logical  logical_function=AND  inputs=2  en=off  latency=0  precision=Full  arith_type=Unsigned  n_bits=16  bin_pt=0  align_bp=on  overflow=[]  quantization=[]  XmcBlockStatus=1  maskContainerNames=tabcontainer1  block_type=logical  block_config=sysgen:Logical_config
  Logical1 : hdlBasic/Logical  logical_function=AND  inputs=3  en=off  latency=0  precision=Full  arith_type=Unsigned  n_bits=16  bin_pt=0  align_bp=on  overflow=[]  quantization=[]  XmcBlockStatus=1  maskContainerNames=tabcontainer1  block_type=logical  block_config=sysgen:Logical_config
  Logical8 : hdlBasic/Logical  logical_function=AND  inputs=2  en=off  latency=0  precision=Full  arith_type=Unsigned  n_bits=16  bin_pt=0  align_bp=on  overflow=[]  quantization=[]  XmcBlockStatus=1  maskContainerNames=tabcontainer1  block_type=logical  block_config=sysgen:Logical_config
  Register : hdlBasic/Register  init=0  rst=on  en=off  XmcBlockStatus=1  maskContainerNames=tabcontainer1  block_type=register  block_config=sysgen:Register_config
  Register1 : hdlBasic/Register  init=0  rst=on  en=off  XmcBlockStatus=1  maskContainerNames=tabcontainer1  block_type=register  block_config=sysgen:Register_config
  Relational : hdlBasic/Relational  mode=a<b  op_type=Bool  en=off  latency=0  XmcBlockStatus=1  maskContainerNames=tabcontainer1  block_type=relational  block_config=sysgen:Relational_config
  Relational8 : hdlBasic/Relational  mode=a<b  op_type=Bool  en=off  latency=0  XmcBlockStatus=1  maskContainerNames=tabcontainer1  block_type=relational  block_config=sysgen:Relational_config
  Terminator : Terminator
  shannonE : Subsystem
      settings: PortSchema="{\"entries\":[{\"content\":{\"sides\":[{\"content\":{\"connectorIds\":[\"In1\",\"In2\",\"Out3\"]},\"type\":\"ConnectorPlacement.EquallySpacedRectSide\",\"uuid\":\"9d039a16-3a48-49d5-80b7-ade04a8e7f96\"},{\"content\":{\"connectorIds\":[\"Out1\",\"Out2\",\"In3\"],\"side\":\"RIGHT\"},\"type\":\"ConnectorPlacement.EquallySpacedRectSide\",\"uuid\":\"bb4be220-296c-4d2d-b90e-a958a467eb47\"},{\"content\":{\"connectorIds\":[],\"side\":\"TOP\"},\"type\":\"ConnectorPlacement.EquallySpacedRectSide\",\"uuid\":\"bb4a24ca-25c4-4b34-8f6b-74df8c85655a\"}]},\"type\":\"ConnectorPlacement.EquallySpacedConnector\",\"uuid\":\"a2ca7259-7cd6-4f5b-b082-7ba40fce56a8\"}],\"packageUris\":[\"http://schema.mathworks.com/mf0/Connector/R2020b\"],\"version\":\"1.0\"}"
  swt_m_data_tdata : hdlBasic/Gateway Out  inherit_from_input=off  hdl_port=on  rows=1  columns=1  UseAsDAC=off  DACChannel='1'  interface=None  automatic_assignment=on  address_offset=hex2dec('00')  intf_name=''  intf_description=''  timing_constraint=None  locs_specified=off  LOCs={}  io_standard={}  XmcBlockStatus=1  maskContainerNames=group4  block_type=gatewayout  block_config=sysgen:gateway_out_config  block_width_w=590  block_height_w=620  block_width=620  block_height=750
  swt_m_data_tvalid : hdlBasic/Gateway Out  inherit_from_input=off  hdl_port=on  rows=1  columns=1  UseAsDAC=off  DACChannel='1'  interface=None  automatic_assignment=on  address_offset=hex2dec('00')  intf_name=''  intf_description=''  timing_constraint=None  locs_specified=off  LOCs={}  io_standard={}  XmcBlockStatus=1  maskContainerNames=group4  block_type=gatewayout  block_config=sysgen:gateway_out_config  block_width_w=590  block_height_w=620  block_width=620  block_height=750
  m_data_tdata : Outport  VectorParamsAs1DForOutWhenUnconnected=off
  m_data_tvalid : Outport  Port=2  VectorParamsAs1DForOutWhenUnconnected=off
  s_data_tready : Outport  Port=3
  wires:
  Level-3/1(m_data_tdata) -> Level-4/1(s_data_tdata)
  Level-4/1(m_data_tdata) -> shannonE/1(s_data_tdata)
  s_data_tvalid/1 -> Inverter/1
  Level-4/3(s_data_tready) -> Level-3/3(m_data_ready)
  Level-2/3(s_data_tready) -> s_data_tready/1
  Level-2/2(m_data_tvalid) -> Level-3/2(s_data_tvalid)
  Level-3/2(m_data_tvalid) -> Level-4/2(s_data_tvalid)
  Level-4/2(m_data_tvalid) -> shannonE/2(s_data_tvalid)
  Delay/1 -> FIR_polyphase_decimator_4/1
  shannonE/2(m_data_tvalid) -> Delay/1
  FIR_polyphase_decimator_4/2 -> Delay1/1, Logical1/2
  swt_m_data_tdata/1 -> m_data_tdata/1
  Absolute/1 -> FIR_polyphase_decimator_4/2
  Inverter/1 -> Level-2/2(s_data_tvalid)
  Level-2/1(m_data_tdata) -> Level-3/1(s_data_tdata)
  Level-3/3(s_data_tready) -> Level-2/3(m_data_tready)
  shannonE/3(s_data_tready) -> Level-4/3(m_data_tready)
  shannonE/1(m_data_tdata) -> Absolute/1
  s_data_tdata/1 -> Level-2/1(data_s_tdata)
  Inverter4/1 -> Counter2/1
  Constant12/1 -> Relational8/2
  Counter2/1 -> Relational8/1
  swt_m_data_tvalid/1 -> m_data_tvalid/1
  Logical8/1 -> Counter2/2, swt_m_data_tvalid/1
  Relational8/1 -> Logical/2
  m_data_ready/1 -> Logical1/1, Logical/1, Inverter4/1
  Logical/1 -> Delay/2, shannonE/3(m_data_tready), Absolute/2, FIR_polyphase_decimator_4/3, Logical8/2
  FIR_polyphase_decimator_4/1 -> Terminator/1
  Counter/1 -> Relational/1
  Logical1/1 -> Counter/1
  Relational/1 -> Register1/2, Register/2, Logical1/3
  Constant/1 -> Relational/2
  FIR_polyphase_decimator_4/3 -> Delay2/1
  Register/1 -> swt_m_data_tdata/1
  Register1/1 -> Logical8/1
  Delay1/1 -> Register1/1
  Delay2/1 -> Register/1
